simulink model "Hatch_open_2017b"  (R2017b)
settings: Solver=VariableStepAuto  StartTime=0.0  StopTime=inf  RelTol=1e-3
settings Model: Creator=shiva  LastModifiedBy=shiva
settings DataIOCC: ReturnWorkspaceOutputs=on
settings DebuggingCC: SFMachineParentedDataDiag=error
settings SFSimCC: SimUseLocalCustomCode=on
settings RTWCC: RTWUseLocalCustomCode=on

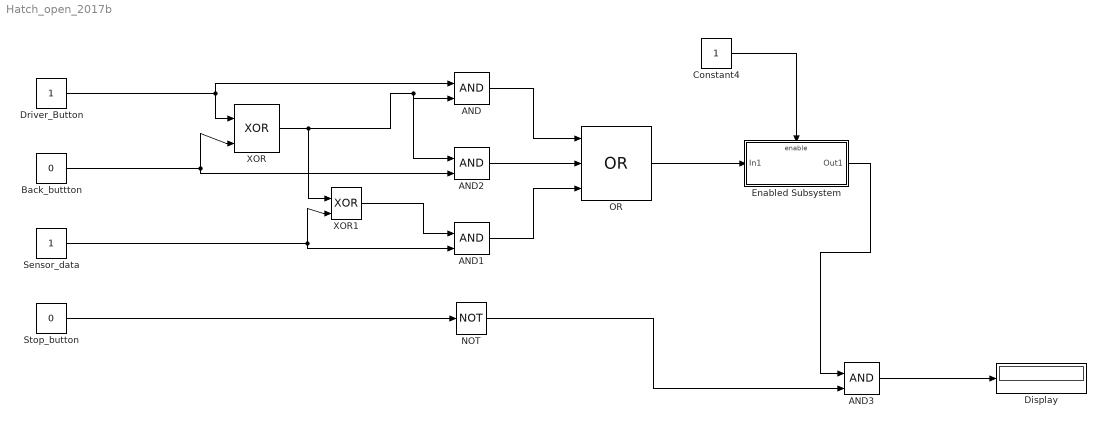
== system Hatch_open_2017b ==
  AND{,1..3} (4 alike) : Logic  IconShape=distinctive  AllPortsSameDT=off  OutDataTypeStr=boolean
  Back_buttton : Constant  Value=0
  Constant4 : Constant
  Display : Display
  Driver_Button : Constant
  Enabled Subsystem : Subsystem  TreatAsAtomicUnit=on
  NOT : Logic  Operator=NOT  IconShape=distinctive  AllPortsSameDT=off  OutDataTypeStr=boolean
  OR : Logic  Operator=OR  Inputs=3  IconShape=distinctive  AllPortsSameDT=off  OutDataTypeStr=boolean
  Sensor_data : Constant
  Stop_button : Constant  Value=0
  XOR : Logic  Operator=XOR  IconShape=distinctive  AllPortsSameDT=off  OutDataTypeStr=boolean
  XOR1 : Logic  Operator=XOR  IconShape=distinctive  AllPortsSameDT=off  OutDataTypeStr=boolean
  wires:
  Driver_Button/1 -> AND/1, XOR/1
  Back_buttton/1 -> AND2/2, XOR/2
  Sensor_data/1 -> AND1/2, XOR1/2
  XOR/1 -> AND2/1, AND/2, XOR1/1
  AND/1 -> OR/1
  AND2/1 -> OR/2
  AND1/1 -> OR/3
  Constant4/1 -> Enabled Subsystem/Enable
  Enabled Subsystem/1(Out1) -> AND3/1
  XOR1/1 -> AND1/1
  OR/1 -> Enabled Subsystem/1(In1)
  AND3/1 -> Display/1
  Stop_button/1 -> NOT/1
  NOT/1 -> AND3/2

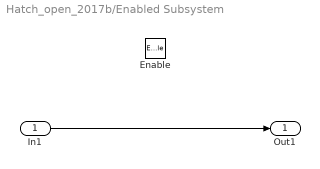
== system Hatch_open_2017b/Enabled Subsystem ==
  In1 : Inport
  Enable : EnablePort
  Out1 : Outport
  wires:
  In1/1 -> Out1/1
